simulink model "AD2ab3_TUN"  (Simulink 4.00)
settings: Solver=ode45  StartTime=0.0  StopTime=100  RelTol=5e-3
libraries: simulink3 x1
settings Model: RTWOptions="-aExtMode=0 -aForceParamTrailComments=0 -aInlineInvariantSignals=0 -aLocalBlockOutputs=0 -aLogVarNameModifier=\"rt_\" -aRTWVerbose=1 -aRollThreshold=5 -aShowEliminatedStatements=1"  OptimizeBlockIOStorage=off  BlockReductionOpt=off

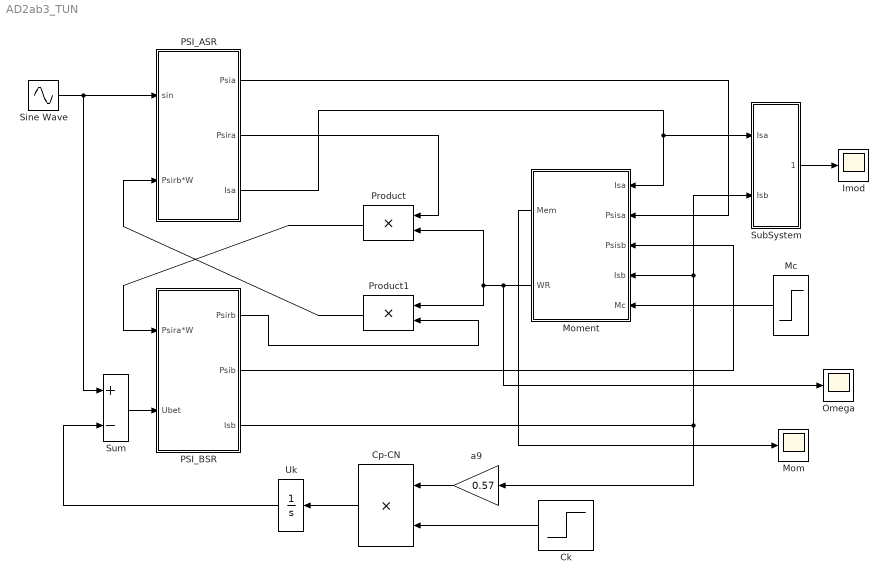
== system AD2ab3_TUN ==
  Ck : Step  Orientation=left  Time=10  Before=0.5  After=1  SampleTime=0
  Cp-CN : Product  Orientation=left  Inputs=2  Multiplication=Element-wise(.*)  SaturateOnIntegerOverflow=on
  Imod : Scope
      settings: TimeRange=auto  YMin=-5  YMax=5  SaveToWorkspace=off  SaveName=ScopeData2  LimitDataPoints=on  MaxDataPoints=5000
  Mc : Step  Orientation=left  Time=5  Before=0  After=0.35  SampleTime=0
  Mom : Scope
      settings: TimeRange=auto  YMin=-5  YMax=5  SaveToWorkspace=off  LimitDataPoints=on  MaxDataPoints=5000
  Moment : Subsystem  Orientation=left
      settings: RTWFcnNameOpts=Auto  RTWFileNameOpts=Auto
  Omega : Scope
      settings: TimeRange=auto  YMin=-0.75  YMax=0.75  SaveToWorkspace=off  SaveName=ScopeData  LimitDataPoints=on  MaxDataPoints=5000
  PSI_ASR : Subsystem
      settings: RTWFcnNameOpts=Auto  RTWFileNameOpts=Auto
  PSI_BSR : Subsystem
      settings: RTWFcnNameOpts=Auto  RTWFileNameOpts=Auto
  Product : Product  Orientation=left  Inputs=2  Multiplication=Element-wise(.*)  SaturateOnIntegerOverflow=on
  Product1 : Product  Orientation=left  Inputs=2  Multiplication=Element-wise(.*)  SaturateOnIntegerOverflow=on
  Sine Wave : Sin  Amplitude=1  Frequency=1  Phase=0  SampleTime=0
  SubSystem : Subsystem
      settings: RTWFcnNameOpts=Auto  RTWFileNameOpts=Auto
  Sum : Sum  Inputs=+-  SaturateOnIntegerOverflow=on
  Uk : Integrator  Orientation=left  ExternalReset=none  InitialConditionSource=internal  InitialCondition=0  LimitOutput=off  UpperSaturationLimit=inf  LowerSaturationLimit=-inf  ShowSaturationPort=off  ShowStatePort=off  AbsoluteTolerance=auto
  a9 : Gain  Orientation=left  Gain=0.57  Multiplication=Element-wise(K.*u)  SaturateOnIntegerOverflow=on
  wires:
  Sine Wave/1 -> PSI_ASR/1(sin), Sum/1
  Mc/1 -> Moment/5(Mc)
  PSI_ASR/1(Psia) -> Moment/2(Psisa)
  PSI_BSR/2(Psib) -> Moment/3(Psisb)
  PSI_BSR/3(Isb) -> a9/1, Moment/4(Isb), SubSystem/2(Isb)
  PSI_ASR/2(Psira) -> Product/1
  PSI_BSR/1(Psirb) -> Product1/2
  Uk/1 -> Sum/2
  Sum/1 -> PSI_BSR/2(Ubet)
  Moment/2(WR) -> Product/2, Product1/1, Omega/1
  Product/1 -> PSI_BSR/1(Psira*W)
  Product1/1 -> PSI_ASR/2(Psirb*W)
  SubSystem/1(Imod) -> Imod/1
  Moment/1(Mem) -> Mom/1
  PSI_ASR/3(Isa) -> Moment/1(Isa), SubSystem/1(Isa)
  a9/1 -> Cp-CN/1
  Cp-CN/1 -> Uk/1
  Ck/1 -> Cp-CN/2

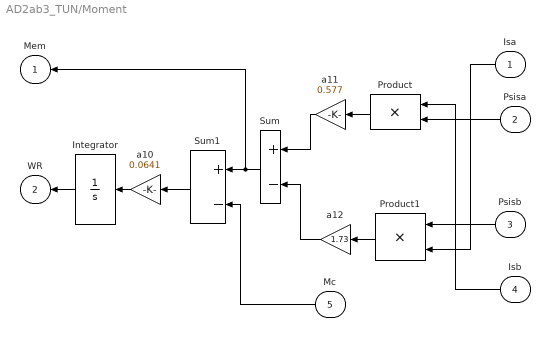
== system AD2ab3_TUN/Moment ==
  Isa : Inport  Orientation=left  Port=1
  Psisa : Inport  Orientation=left  Port=2
  Psisb : Inport  Orientation=left  Port=3
  Isb : Inport  Orientation=left  Port=4
  Mc : Inport  Orientation=left  Port=5
  Integrator : Integrator  Orientation=left  ExternalReset=none  InitialConditionSource=internal  InitialCondition=0  LimitOutput=off  UpperSaturationLimit=inf  LowerSaturationLimit=-inf  ShowSaturationPort=off  ShowStatePort=off  AbsoluteTolerance=auto
  Product : Product  Orientation=left  Inputs=2  Multiplication=Element-wise(.*)  SaturateOnIntegerOverflow=on
  Product1 : Product  Orientation=left  Inputs=2  Multiplication=Element-wise(.*)  SaturateOnIntegerOverflow=on
  Sum : Sum  Orientation=left  Inputs=+-  SaturateOnIntegerOverflow=on
  Sum1 : Sum  Orientation=left  Inputs=+-  SaturateOnIntegerOverflow=on
  a10 : Gain  Orientation=left  Gain=0.0641  Multiplication=Element-wise(K.*u)  SaturateOnIntegerOverflow=on
  a11 : Gain  Orientation=left  Gain=0.577  Multiplication=Element-wise(K.*u)  SaturateOnIntegerOverflow=on
  a12 : Gain  Orientation=left  Gain=1.73  Multiplication=Element-wise(K.*u)  SaturateOnIntegerOverflow=on
  Mem : Outport  Orientation=left  Port=1
  WR : Outport  Orientation=left  Port=2
  wires:
  Psisa/1 -> Product/2
  Psisb/1 -> Product1/1
  Product1/1 -> a12/1
  a12/1 -> Sum/2
  Product/1 -> a11/1
  Mc/1 -> Sum1/2
  Sum/1 -> Sum1/1, Mem/1
  a11/1 -> Sum/1
  Integrator/1 -> WR/1
  Sum1/1 -> a10/1
  a10/1 -> Integrator/1
  Isb/1 -> Product/1
  Isa/1 -> Product1/2

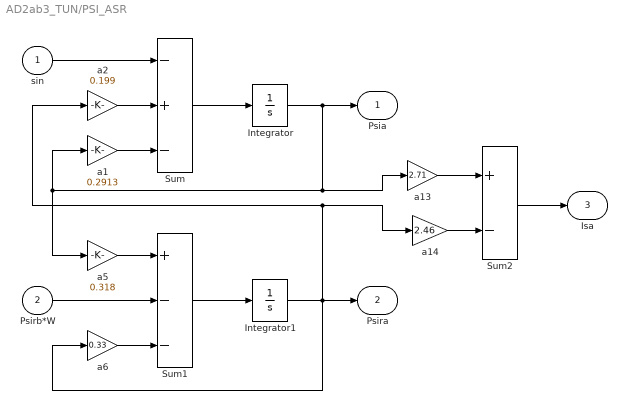
== system AD2ab3_TUN/PSI_ASR ==
  sin : Inport  Port=1
  Psirb*W : Inport  Port=2
  Integrator : Integrator  ExternalReset=none  InitialConditionSource=internal  InitialCondition=0  LimitOutput=off  UpperSaturationLimit=inf  LowerSaturationLimit=-inf  ShowSaturationPort=off  ShowStatePort=off  AbsoluteTolerance=auto
  Integrator1 : Integrator  ExternalReset=none  InitialConditionSource=internal  InitialCondition=0  LimitOutput=off  UpperSaturationLimit=inf  LowerSaturationLimit=-inf  ShowSaturationPort=off  ShowStatePort=off  AbsoluteTolerance=auto
  Sum : Sum  Inputs=-+-  SaturateOnIntegerOverflow=on
  Sum1 : Sum  Inputs=+--  SaturateOnIntegerOverflow=on
  Sum2 : Sum  Inputs=+-  SaturateOnIntegerOverflow=on
  a1 : Gain  Gain=0.2913  Multiplication=Element-wise(K.*u)  SaturateOnIntegerOverflow=on
  a13 : Gain  Gain=2.71  Multiplication=Element-wise(K.*u)  SaturateOnIntegerOverflow=on
  a14 : Gain  Gain=2.46  Multiplication=Element-wise(K.*u)  SaturateOnIntegerOverflow=on
  a2 : Gain  Gain=0.199  Multiplication=Element-wise(K.*u)  SaturateOnIntegerOverflow=on
  a5 : Gain  Gain=0.318  Multiplication=Element-wise(K.*u)  SaturateOnIntegerOverflow=on
  a6 : Gain  Gain=0.33  Multiplication=Element-wise(K.*u)  SaturateOnIntegerOverflow=on
  Psia : Outport  Port=1
  Psira : Outport  Port=2
  Isa : Outport  Port=3
  wires:
  Sum/1 -> Integrator/1
  Integrator/1 -> Psia/1, a1/1, a5/1, a13/1
  a1/1 -> Sum/3
  sin/1 -> Sum/1
  a2/1 -> Sum/2
  Integrator1/1 -> Psira/1, a6/1, a2/1, a14/1
  Sum1/1 -> Integrator1/1
  a6/1 -> Sum1/3
  Psirb*W/1 -> Sum1/2
  a5/1 -> Sum1/1
  a13/1 -> Sum2/1
  a14/1 -> Sum2/2
  Sum2/1 -> Isa/1

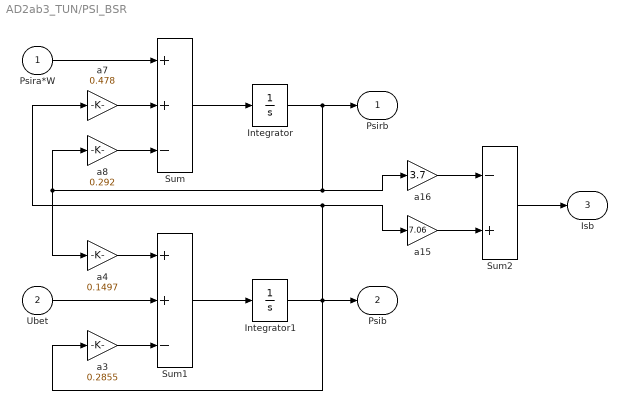
== system AD2ab3_TUN/PSI_BSR ==
  Psira*W : Inport  Port=1
  Ubet : Inport  Port=2
  Integrator : Integrator  ExternalReset=none  InitialConditionSource=internal  InitialCondition=0  LimitOutput=off  UpperSaturationLimit=inf  LowerSaturationLimit=-inf  ShowSaturationPort=off  ShowStatePort=off  AbsoluteTolerance=auto
  Integrator1 : Integrator  ExternalReset=none  InitialConditionSource=internal  InitialCondition=0  LimitOutput=off  UpperSaturationLimit=inf  LowerSaturationLimit=-inf  ShowSaturationPort=off  ShowStatePort=off  AbsoluteTolerance=auto
  Sum : Sum  Inputs=++-  SaturateOnIntegerOverflow=on
  Sum1 : Sum  Inputs=++-  SaturateOnIntegerOverflow=on
  Sum2 : Sum  Inputs=-+  SaturateOnIntegerOverflow=on
  a15 : Gain  Gain=7.06  Multiplication=Element-wise(K.*u)  SaturateOnIntegerOverflow=on
  a16 : Gain  Gain=3.7  Multiplication=Element-wise(K.*u)  SaturateOnIntegerOverflow=on
  a3 : Gain  Gain=0.2855  Multiplication=Element-wise(K.*u)  SaturateOnIntegerOverflow=on
  a4 : Gain  Gain=0.1497  Multiplication=Element-wise(K.*u)  SaturateOnIntegerOverflow=on
  a7 : Gain  Gain=0.478  Multiplication=Element-wise(K.*u)  SaturateOnIntegerOverflow=on
  a8 : Gain  Gain=0.292  Multiplication=Element-wise(K.*u)  SaturateOnIntegerOverflow=on
  Psirb : Outport  Port=1
  Psib : Outport  Port=2
  Isb : Outport  Port=3
  wires:
  Sum2/1 -> Isb/1
  a15/1 -> Sum2/2
  a16/1 -> Sum2/1
  a4/1 -> Sum1/1
  Ubet/1 -> Sum1/2
  a3/1 -> Sum1/3
  Sum1/1 -> Integrator1/1
  Integrator1/1 -> a15/1, a7/1, a3/1, Psib/1
  a7/1 -> Sum/2
  Psira*W/1 -> Sum/1
  a8/1 -> Sum/3
  Integrator/1 -> a16/1, a4/1, a8/1, Psirb/1
  Sum/1 -> Integrator/1

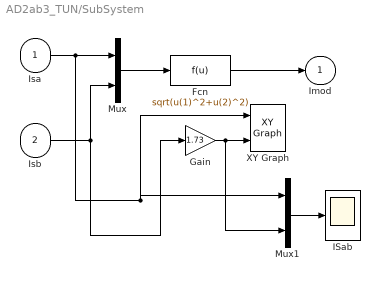
== system AD2ab3_TUN/SubSystem ==
  Isa : Inport  Port=1
  Isb : Inport  Port=2
  Fcn : Fcn  Expr=sqrt(u(1)^2+u(2)^2)
  Gain : Gain  Gain=1.73  Multiplication=Element-wise(K.*u)  SaturateOnIntegerOverflow=on
  ISab : Scope
      settings: TimeRange=50  YMin=-3e+006  YMax=250000  SaveToWorkspace=off  SaveName=ScopeData4  LimitDataPoints=on  MaxDataPoints=5000
  Mux : Mux  Inputs=2
  Mux1 : Mux  Inputs=2
  XY Graph : simulink3/Sinks/XY Graph  xmin=-12  xmax=12  ymin=-12  ymax=12  st=-1
  Imod : Outport  Port=1
  wires:
  Isa/1 -> Mux/1, XY Graph/1, Mux1/1
  Isb/1 -> Mux/2, Gain/1
  Mux/1 -> Fcn/1
  Fcn/1 -> Imod/1
  Mux1/1 -> ISab/1
  Gain/1 -> XY Graph/2, Mux1/2
